simulink model "mtv1"  (R2015b)
settings: Solver=FixedStepDiscrete  SolverMode=SingleTasking  StartTime=0.0  StopTime=sim_stop_time  FixedStep=sim_time_step_size  RelTol=1e-3
PreLoadFcn:
  | nimbus_bus_all;
  | mtv_bus_all;
undefined symbols (not defined in the file or in its folder): csc_sim_mtv_simulation, csc_sim_mtv_simulation_lib, csci_gsse_mtv, csci_gsse_mtv_lib, csu_tfm_tether_mtv, ini_epoch_seconds, sim_time_step_size, swm_num_switches, tfm_attachment_location_body, tfm_cg_enable, tfm_forces_enable, tfm_hanging_location_topo, tfm_horseshoe_bolt_mass, tfm_moments_enable, tfm_sleeve_mass, tfm_tether_mass_per_length, tfm_tether_spring_constant, tfm_tether_unstretched_length
libraries: util_common_lib x8, util_info_lib x2, simulink x2, util_quat_lib x2, csci_fsw_mtv_lib x1, csc_gnd_sta_lib x1, telem_conversion_lib x1, csc_egt_egc_thruster_lib x1, csc_enf_environmental_forces_mtv_lib x1, csc_prs_pressure_system_sim_lib x1, csc_pwr_power_system_sim_lib x1, csc_rigid_body_dynamics_lib x1
settings Model: ExtModeTrigDuration=100  Creator=ianmga  LastModifiedBy=jimkaidy
settings DataIOCC: LimitDataPoints=off  SaveFormat=Array  SaveOutput=off  SaveTime=off  StateSaveName=tmp_raccel_xout  SignalLoggingName=raw_event_logs
settings OptimizationCC: ExpressionDepthLimit=2147483647  InitFltsAndDblsToZero=on  OptimizeModelRefInitCode=on
settings DebuggingCC: CheckSSInitialOutputMsg=off  UnderspecifiedInitializationDetection=Classic  MergeDetectMultiDrivingBlocksExec=none  SolverPrmCheckMsg=warning  UnderSpecifiedDataTypeMsg=warning  FcnCallInpInsideContextMsg=UseLocalSettings  BusObjectLabelMismatch=error  StateNameClashWarn=warning  StrictBusMsg=WarnOnBusTreatedAsVector
settings HardwareCC: ProdBitPerPointer=32  ProdLargestAtomicFloat=None  ProdIntDivRoundTo=Undefined  ProdEndianess=Unspecified  ProdWordSize=32  ProdHWDeviceType=32-bit Generic  TargetHWDeviceType=32-bit Generic
settings SFSimCC: SimParseCustomCode=off
settings SFSimCC: SimUserIncludeDirs=|
  | ../sim/fhw/sensors/cameras/kir
  | ../fsw/est/kcv
  | ../fsw/est/kfd
  | ../externals/minopencv/include
settings RTWCC: SystemTargetFile=ert.tlc  GenCodeOnly=on  TemplateMakefile=ert_default_tmf  Description=Embedded Coder  RetainRTWFile=on  RTWUseSimCustomCode=on
settings RTWCC: CustomInclude=|
  | ../sim/fhw/sensors/cameras/kir
  | ../fsw/est/kcv
  | ../fsw/est/kfd
  | ../externals/minopencv/include
settings CodeAppCC: ForceParamTrailComments=on  IgnoreCustomStorageClasses=off  MaxIdLength=128  SimulinkDataObjDesc=on  SFDataObjDesc=on  MangleLength=10  CustomSymbolStrType=$N$R$M  InsertBlockDesc=on  InternalIdentifier=Classic  ReqsInCode=on
settings ERTTargetCC: GenerateSampleERTMain=on  MultiInstanceERTCode=on  CodeInterfacePackaging=Reusable function  RootIOFormat=Structure reference  ERTCustomFileTemplate=csl_interface.tlc
settings ConfigComp: CovModelRefEnable=Off  CovSFcnEnable=off

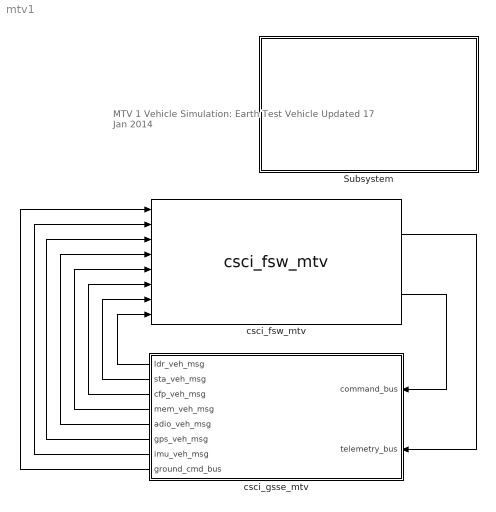
== system mtv1 ==
  note: MTV 1 Vehicle Simulation: Earth Test Vehicle
      |
      | Updated 17 Jan 2014
  Subsystem : Subsystem
      mask Display: image('nimbus2.png')
  csci_fsw_mtv : csci_fsw_mtv_lib/csci_fsw_mtv
  csci_gsse_mtv : Subsystem  AncestorBlock=csci_gsse_mtv_lib/csci_gsse_mtv
  wires:
  csci_fsw_mtv/1 -> csci_gsse_mtv/2(telemetry_bus)
  csci_gsse_mtv/2(sta_veh_msg) -> csci_fsw_mtv/7
  csci_fsw_mtv/2 -> csci_gsse_mtv/1(command_bus)
  csci_gsse_mtv/1(ldr_veh_msg) -> csci_fsw_mtv/8
  csci_gsse_mtv/3(cfp_veh_msg) -> csci_fsw_mtv/6
  csci_gsse_mtv/4(mem_veh_msg) -> csci_fsw_mtv/5
  csci_gsse_mtv/5(adio_veh_msg) -> csci_fsw_mtv/4
  csci_gsse_mtv/6(gps_veh_msg) -> csci_fsw_mtv/3
  csci_gsse_mtv/8(ground_cmd_bus) -> csci_fsw_mtv/1
  csci_gsse_mtv/7(imu_veh_msg) -> csci_fsw_mtv/2

== system mtv1/Subsystem ==

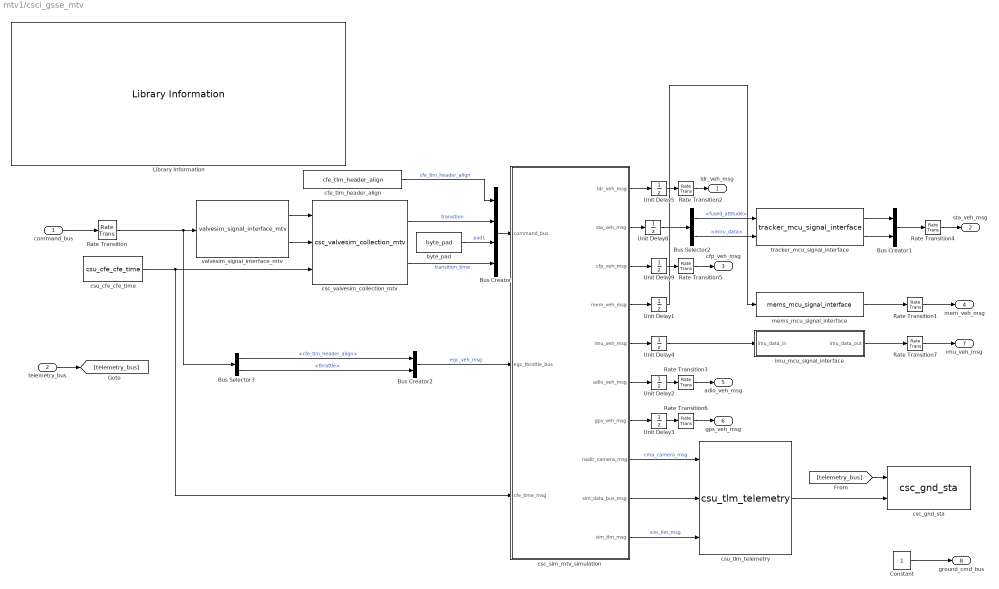
== system mtv1/csci_gsse_mtv ==
  command_bus : Inport
  telemetry_bus : Inport  Port=2
  Bus Creator : BusCreator  Inputs=4  OutDataTypeStr=Bus: thr_sim_msg  NonVirtualBus=on
  Bus Creator2 : BusCreator  Inputs=2  OutDataTypeStr=Bus: egc_veh_msg  NonVirtualBus=on
  Bus Selector2 : BusSelector  OutputSignals=fused_attitude,miru_data
  Bus Selector3 : BusSelector  OutputSignals=egc_bus_msg.cfe_tlm_header_align,egc_bus_msg.throttle
  Bus Creator1 : BusCreator  Inputs=2
  Constant : Constant
  Library Information : util_info_lib/Library Information  owner='NONE'
  Rate Transition{,1..7} (8 alike) : RateTransition  Integrity=off
  Unit Delay{1..5,8..9} (7 alike) : UnitDelay  SampleTime=-1
  byte_pad : util_common_lib/byte_pad  n_bytes=6
  cfe_tlm_header_align : util_common_lib/cfe_tlm_header_align
  csc_gnd_sta : csc_gnd_sta_lib/csc_gnd_sta  dir_name=scenario_data_dir
  csc_sim_mtv_simulation : Subsystem  Tag=GSSE; MDL_TICK=THR_SIM_MSG  AncestorBlock=csc_sim_mtv_simulation_lib/csc_sim_mtv_simulation  TreatAsAtomicUnit=on  SystemSampleTime=sim_time_step_size
  csc_valvesim_collection_mtv : csc_valvesim_collection_mtv_lib/csc_valvesim_collection_mtv  SystemSampleTime=-1
  csu_cfe_cfe_time : csu_cfe_cfe_time_lib/csu_cfe_cfe_time  sch_dt=sim_time_step_size
  csu_tlm_telemetry : csu_tlm_telemetry_lib/csu_tlm_telemetry  num_inputs=3  output_bus_name=sim_telemetry_bus_msg
  imu_mcu_signal_interface : Subsystem
  mems_mcu_signal_interface : csu_mems_mcu_signal_interface_lib/mems_mcu_signal_interface
  tracker_mcu_signal_interface : csu_tracker_mcu_signal_interface_lib/tracker_mcu_signal_interface
  valvesim_signal_interface_mtv : csu_valvesim_signal_interface_mtv_lib/valvesim_signal_interface_mtv
  ldr_veh_msg : Outport
  sta_veh_msg : Outport  Port=2
  cfp_veh_msg : Outport  Port=3
  mem_veh_msg : Outport  Port=4
  adio_veh_msg : Outport  Port=5
  gps_veh_msg : Outport  Port=6
  imu_veh_msg : Outport  Port=7
  ground_cmd_bus : Outport  Port=8
  wires:
  telemetry_bus/1 -> [telemetry_bus]
  csc_sim_mtv_simulation/9(sim_data_bus_msg) -> csu_tlm_telemetry/2
  Unit Delay9/1 -> Rate Transition5/1
  Unit Delay5/1 -> Rate Transition2/1
  csc_sim_mtv_simulation/1(ldr_veh_msg) -> Unit Delay5/1
  csc_sim_mtv_simulation/3(cfp_veh_msg) -> Unit Delay9/1
  Constant/1 -> ground_cmd_bus/1
  command_bus/1 -> Rate Transition/1
  Rate Transition2/1 -> ldr_veh_msg/1
  Rate Transition4/1 -> sta_veh_msg/1
  Rate Transition5/1 -> cfp_veh_msg/1
  csc_sim_mtv_simulation/2(sta_veh_msg) -> Unit Delay8/1
  csc_sim_mtv_simulation/8(nadir_camera_msg) -> csu_tlm_telemetry/1  "cma_camera_msg"
  csc_sim_mtv_simulation/10(sim_tlm_msg) -> csu_tlm_telemetry/3  "sim_tlm_msg"
  csu_tlm_telemetry/1 -> csc_gnd_sta/2
  [telemetry_bus] -> csc_gnd_sta/1
  valvesim_signal_interface_mtv/1 -> csc_valvesim_collection_mtv/1
  csc_valvesim_collection_mtv/1 -> Bus Creator/2  "transition"
  csc_valvesim_collection_mtv/2 -> Bus Creator/4  "transition_time"
  Bus Creator/1 -> csc_sim_mtv_simulation/1(command_bus)
  csu_cfe_cfe_time/1 -> csc_sim_mtv_simulation/3(cfe_time_msg), csc_valvesim_collection_mtv/3
  byte_pad/1 -> Bus Creator/3  "pad1"
  Rate Transition/1 -> Bus Selector3/1, valvesim_signal_interface_mtv/1
  Bus Creator2/1 -> csc_sim_mtv_simulation/2(egc_throttle_bus)  "egc_veh_msg"
  cfe_tlm_header_align/1 -> Bus Creator/1  "cfe_tlm_header_align"
  valvesim_signal_interface_mtv/2 -> csc_valvesim_collection_mtv/2
  Bus Creator1/1 -> Rate Transition4/1
  tracker_mcu_signal_interface/2 -> Bus Creator1/2
  tracker_mcu_signal_interface/1 -> Bus Creator1/1
  Bus Selector2/2 -> tracker_mcu_signal_interface/2  "<miru_data>"
  Bus Selector2/1 -> tracker_mcu_signal_interface/1  "<fused_attitude>"
  Unit Delay8/1 -> Bus Selector2/1
  csc_sim_mtv_simulation/4(mem_veh_msg) -> Unit Delay1/1
  Unit Delay1/1 -> mems_mcu_signal_interface/1
  Rate Transition1/1 -> mem_veh_msg/1
  mems_mcu_signal_interface/1 -> Rate Transition1/1
  Bus Selector3/1 -> Bus Creator2/1  "<cfe_tlm_header_align>"
  Bus Selector3/2 -> Bus Creator2/2  "<throttle>"
  Unit Delay2/1 -> Rate Transition3/1
  csc_sim_mtv_simulation/6(adio_veh_msg) -> Unit Delay2/1
  Rate Transition3/1 -> adio_veh_msg/1
  Unit Delay3/1 -> Rate Transition6/1
  Rate Transition6/1 -> gps_veh_msg/1
  csc_sim_mtv_simulation/7(gps_veh_msg) -> Unit Delay3/1
  csc_sim_mtv_simulation/5(imu_veh_msg) -> Unit Delay4/1
  Unit Delay4/1 -> imu_mcu_signal_interface/1(imu_data_in)
  Rate Transition7/1 -> imu_veh_msg/1
  imu_mcu_signal_interface/1(imu_data_out) -> Rate Transition7/1

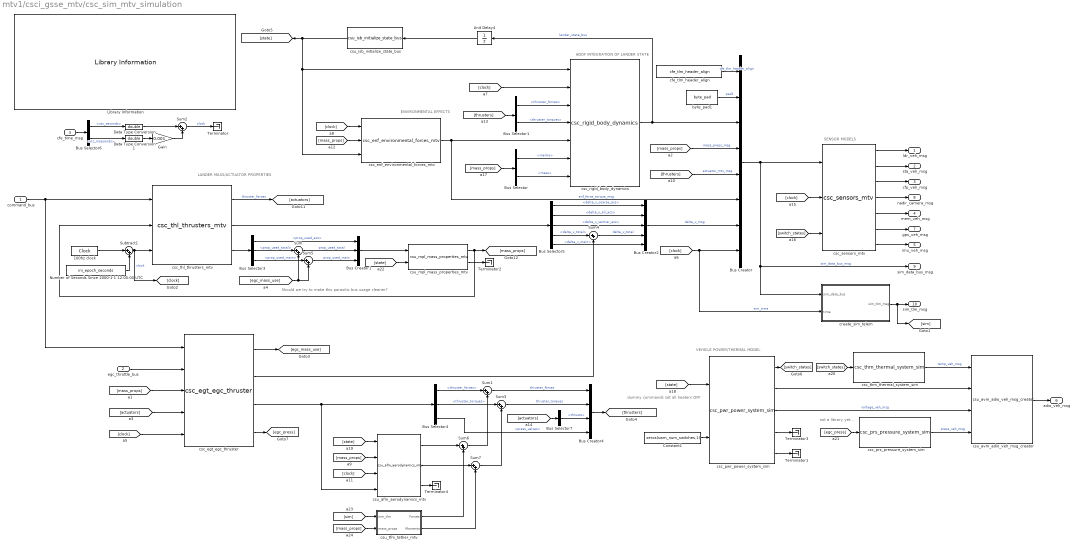
== system mtv1/csci_gsse_mtv/csc_sim_mtv_simulation ==
  note: not a library yet....
  note: VEHICLE POWER/THERMAL MODEL
  note: dummy commands set all heaters OFF
  note: LANDER MASS/ACTUATOR PROPERTIES
  note: 6DOF INTEGRATION OF LANDER STATE
  note: ENVIRONMENTAL EFFECTS
  note: SENSOR MODELS
  note: Should we try to make this parasitic bus usage cleaner?
  command_bus : Inport
  egc_throttle_bus : Inport  Port=2
  cfe_time_msg : Inport  Port=3  OutDataTypeStr=Bus: cfe_time_msg
  100hz clock : DigitalClock  SampleTime=sim_time_step_size
  Bus Creator : BusCreator  Inputs=8  OutDataTypeStr=Bus: sim_data_mtv_msg  NonVirtualBus=on
  Bus Creator1 : BusCreator  Inputs=3
  Bus Creator2 : BusCreator  Inputs=5
  Bus Creator4 : BusCreator  Inputs=4  OutDataTypeStr=Bus: actuator_mtv_msg_t
  Bus Selector : BusSelector  OutputSignals=inertia,mass
  Bus Selector1 : BusSelector  OutputSignals=thruster_forces,thruster_torques
  Bus Selector3 : BusSelector  OutputSignals=prop_used_acs,prop_used_total,prop_used_main
  Bus Selector4 : BusSelector  OutputSignals=thruster_forces,thruster_torques,press_valves
  Bus Selector5 : BusSelector  OutputSignals=delta_v_coarse_acs,delta_v_all_acs,delta_v_vernier_acs,delta_v_total,delta_v_main
  Bus Selector6 : BusSelector  OutputSignals=utc_seconds,utc_mseconds
  Bus Selector7 : BusSelector  OutputSignals=thrusts
  Constant1 : Constant  Value=zeros(swm_num_switches,1)  OutDataTypeStr=double
  Data Type Conversion : DataTypeConversion  OutDataTypeStr=double
  Data Type Conversion1 : DataTypeConversion  OutDataTypeStr=double
  Gain : Gain  Gain=0.001
  Library Information : util_info_lib/Library Information  owner='NONE'
  Number of Seconds Since 2000-1-1 12:00:00 UTC : Constant  Description=|  Value=ini_epoch_seconds
      | Number of Seconds                   
      | July 4, 2014 22:40:00 UTC           
      | Calculate on Web Site:              
      | www.mbari.org/staff/rich/utccalc.htm
  Subtract1 : Sum  Inputs=|++
  Sum{,1..7} (8 alike) : Sum  Inputs=|++
  Terminator{,1..4} (5 alike) : Terminator
  Unit Delay4 : UnitDelay  SampleTime=-1
  byte_pad1 : util_common_lib/byte_pad  n_bytes=4
  cfe_tlm_header_align : util_common_lib/cfe_tlm_header_align
  create_sim_telem : Subsystem
  csc_egt_egc_thruster : csc_egt_egc_thruster_lib/csc_egt_egc_thruster
  csc_enf_environmental_forces_mtv : csc_enf_environmental_forces_mtv_lib/csc_enf_environmental_forces_mtv
  csc_prs_pressure_system_sim : csc_prs_pressure_system_sim_lib/csc_prs_pressure_system_sim
  csc_pwr_power_system_sim : csc_pwr_power_system_sim_lib/csc_pwr_power_system_sim
  csc_rigid_body_dynamics : csc_rigid_body_dynamics_lib/csc_rigid_body_dynamics
  csc_sensors_mtv : csc_sensors_mtv_lib/csc_sensors_mtv
  csc_thl_thrusters_mtv : csc_thl_thrusters_mtv_lib/csc_thl_thrusters_mtv
  csc_thm_thermal_system_sim : csc_thm_thermal_system_sim_lib/csc_thm_thermal_system_sim
  csu_afm_aerodynamics_mtv : csu_afm_aerodynamics_lib/csu_afm_aerodynamics_mtv  SystemSampleTime=-1
  csu_avm_adio_veh_msg_creator : csu_avm_adio_veh_msg_creator_lib/csu_avm_adio_veh_msg_creator
  csu_isb_initialize_state_bus : csu_isb_initialize_state_bus_lib/csu_isb_initialize_state_bus
  csu_mpl_mass_properties_mtv : csu_mpl_mass_properties_mtv_lib/csu_mpl_mass_properties_mtv
  csu_tfm_tether_mtv : Subsystem  AncestorBlock=csu_tfm_tether_mtv/csu_tfm_tether_mtv
  ldr_veh_msg : Outport
  sta_veh_msg : Outport  Port=2
  cfp_veh_msg : Outport  Port=3
  mem_veh_msg : Outport  Port=4
  imu_veh_msg : Outport  Port=5
  adio_veh_msg : Outport  Port=6
  gps_veh_msg : Outport  Port=7
  nadir_camera_msg : Outport  Port=8
  sim_data_bus_msg : Outport  Port=9
  sim_tlm_msg : Outport  Port=10
  wires:
  csu_afm_aerodynamics_mtv/3 -> Terminator4/1
  [clock] -> csu_afm_aerodynamics_mtv/3
  Sum3/1 -> Bus Creator4/2  "thruster_torques"
  Bus Selector7/1 -> Bus Creator4/3  "<thrusts>"
  [actuators] -> Bus Selector7/1
  Bus Creator4/1 -> [thrusters]
  Sum1/1 -> Bus Creator4/1  "thruster_forces"
  csc_egt_egc_thruster/3 -> Bus Selector4/1, csu_afm_aerodynamics_mtv/4
  [switch_states] -> csc_sensors_mtv/3
  csc_pwr_power_system_sim/5 -> Terminator1/1
  csc_pwr_power_system_sim/4 -> Terminator3/1
  csc_pwr_power_system_sim/1 -> [switch_states]
  [state] -> csc_pwr_power_system_sim/1
  Constant1/1 -> csc_pwr_power_system_sim/2
  [clock] -> csc_sensors_mtv/2
  Unit Delay4/1 -> csu_isb_initialize_state_bus/1
  csu_isb_initialize_state_bus/1 -> csc_enf_environmental_forces_mtv/3, csc_rigid_body_dynamics/1, [state]
  [clock] -> csc_rigid_body_dynamics/2
  cfe_tlm_header_align/1 -> Bus Creator/1  "cfe_tlm_header_align"
  csc_sensors_mtv/4 -> nadir_camera_msg/1
  csc_sensors_mtv/3 -> cfp_veh_msg/1
  csc_sensors_mtv/2 -> sta_veh_msg/1
  csc_sensors_mtv/1 -> ldr_veh_msg/1
  Bus Selector6/1 -> Data Type Conversion/1  "<utc_seconds>"
  Gain/1 -> Sum2/2
  Data Type Conversion1/1 -> Gain/1
  Data Type Conversion/1 -> Sum2/1
  Bus Selector6/2 -> Data Type Conversion1/1  "<utc_mseconds>"
  cfe_time_msg/1 -> Bus Selector6/1
  egc_throttle_bus/1 -> csc_egt_egc_thruster/2
  [mass_props] -> csc_egt_egc_thruster/3
  [actuators] -> csc_egt_egc_thruster/4
  Bus Selector5/1 -> Bus Creator2/1  "<delta_v_coarse_acs>"
  Bus Selector5/2 -> Bus Creator2/2  "<delta_v_all_acs>"
  Bus Selector5/3 -> Bus Creator2/3  "<delta_v_vernier_acs>"
  Bus Selector5/5 -> Bus Creator2/5  "<delta_v_main>"
  Sum4/1 -> Bus Creator2/4  "delta_v_total"
  Bus Selector5/4 -> Sum4/1  "<delta_v_total>"
  csc_thl_thrusters_mtv/2 -> Bus Selector5/1
  Bus Creator2/1 -> Bus Creator/7  "delta_v_msg"
  csc_egt_egc_thruster/2 -> Sum4/2
  Bus Creator1/1 -> csu_mpl_mass_properties_mtv/1
  Bus Selector3/3 -> Sum5/1  "<prop_used_main>"
  Bus Selector3/1 -> Bus Creator1/1  "<prop_used_acs>"
  Sum/1 -> Bus Creator1/2  "prop_used_total"
  [egc_mass_use] -> Sum5/2, Sum/2
  Bus Selector3/2 -> Sum/1  "<prop_used_total>"
  csc_egt_egc_thruster/1 -> [egc_mass_use]
  csc_thl_thrusters_mtv/3 -> Bus Selector3/1
  byte_pad1/1 -> Bus Creator/2  "pad1"
  Subtract1/1 -> [clock], csc_thl_thrusters_mtv/3  "clock"
  [clock] -> Bus Creator/8, create_sim_telem/2(time)  "sim_time"
  create_sim_telem/1(sim_tlm_msg) -> [sim], sim_tlm_msg/1
  Bus Creator/1 -> create_sim_telem/1(sim_data_bus), sim_data_bus_msg/1, csc_sensors_mtv/1  "sim_data_bus_msg"
  csc_rigid_body_dynamics/1 -> Unit Delay4/1, Bus Creator/3  "lander_state_bus"
  [mass_props] -> Bus Selector/1
  [thrusters] -> Bus Selector1/1
  [thrusters] -> Bus Creator/5  "actuator_mtv_msg"
  [mass_props] -> Bus Creator/4  "mass_props_msg"
  Bus Selector/2 -> csc_rigid_body_dynamics/7  "<mass>"
  Bus Selector/1 -> csc_rigid_body_dynamics/6  "<inertia>"
  csu_mpl_mass_properties_mtv/1 -> csc_thl_thrusters_mtv/2, [mass_props]
  Bus Selector1/1 -> csc_rigid_body_dynamics/3  "<thruster_forces>"
  Bus Selector1/2 -> csc_rigid_body_dynamics/4  "<thruster_torques>"
  csc_enf_environmental_forces_mtv/1 -> csc_rigid_body_dynamics/5, Bus Creator/6  "enf_force_torque_msg"
  csc_thl_thrusters_mtv/1 -> [actuators]  "thruster_forces"
  [clock] -> csc_enf_environmental_forces_mtv/1
  [mass_props] -> csc_enf_environmental_forces_mtv/2
  csc_sensors_mtv/5 -> mem_veh_msg/1
  Number of Seconds Since 2000-1-1 12:00:00 UTC/1 -> Subtract1/2
  100hz clock/1 -> Subtract1/1
  Sum2/1 -> Terminator/1  "clock"
  [switch_states] -> csc_thm_thermal_system_sim/1
  csu_avm_adio_veh_msg_creator/1 -> adio_veh_msg/1
  csc_thm_thermal_system_sim/1 -> csu_avm_adio_veh_msg_creator/1  "temp_veh_msg"
  csc_pwr_power_system_sim/2 -> csu_avm_adio_veh_msg_creator/2
  csc_pwr_power_system_sim/3 -> csu_avm_adio_veh_msg_creator/3  "voltage_veh_msg"
  [egc_press] -> csc_prs_pressure_system_sim/1
  csc_prs_pressure_system_sim/1 -> csu_avm_adio_veh_msg_creator/4  "press_veh_msg"
  csc_egt_egc_thruster/4 -> [egc_press]
  command_bus/1 -> csc_egt_egc_thruster/1, csc_thl_thrusters_mtv/1
  [clock] -> csc_egt_egc_thruster/5
  Sum5/1 -> Bus Creator1/3  "prop_used_main"
  Bus Selector4/3 -> Bus Creator4/4  "<press_valves>"
  csu_mpl_mass_properties_mtv/2 -> Terminator2/1
  csc_sensors_mtv/6 -> gps_veh_msg/1
  [state] -> csu_mpl_mass_properties_mtv/2
  csc_sensors_mtv/7 -> imu_veh_msg/1
  [mass_props] -> csu_afm_aerodynamics_mtv/2
  [state] -> csu_afm_aerodynamics_mtv/1
  Bus Selector4/1 -> Sum1/1  "<thruster_forces>"
  Bus Selector4/2 -> Sum3/1  "<thruster_torques>"
  [mass_props] -> csu_tfm_tether_mtv/2(mass_props)
  [sim] -> csu_tfm_tether_mtv/1(sim_tlm)
  csu_afm_aerodynamics_mtv/1 -> Sum6/1
  csu_tfm_tether_mtv/1(Forces) -> Sum6/2
  csu_afm_aerodynamics_mtv/2 -> Sum7/1
  csu_tfm_tether_mtv/2(Moments) -> Sum7/2
  Sum6/1 -> Sum1/2
  Sum7/1 -> Sum3/2

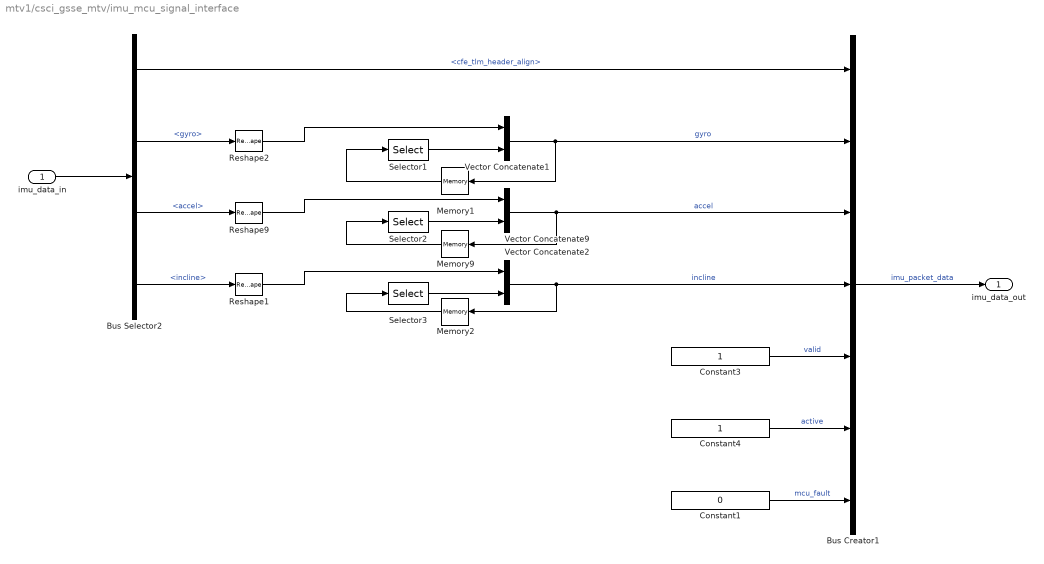
== system mtv1/csci_gsse_mtv/imu_mcu_signal_interface ==
  imu_data_in : Inport
  Bus Selector2 : BusSelector  OutputSignals=cfe_tlm_header_align,gyro,accel,incline
  Bus Creator1 : BusCreator  Inputs=7
  Constant1 : Constant  Value=0  OutDataTypeStr=uint8
  Constant3 : Constant  OutDataTypeStr=uint16
  Constant4 : Constant  OutDataTypeStr=uint8
  Memory1 : Memory  X0=zeros(10,3)  InheritSampleTime=on
  Memory2 : Memory  X0=zeros(10,3)  InheritSampleTime=on
  Memory9 : Memory  X0=zeros(10,3)  InheritSampleTime=on
  Reshape1 : Reshape  OutputDimensionality=Row vector (2-D)
  Reshape2 : Reshape  OutputDimensionality=Row vector (2-D)
  Reshape9 : Reshape  OutputDimensionality=Row vector (2-D)
  Selector1 : Selector  NumberOfDimensions=2  InputPortWidth=10  IndexOptions=Index vector (dialog),Select all  Indices=[1:9],1  OutputSizes=1,1
  Selector2 : Selector  NumberOfDimensions=2  InputPortWidth=10  IndexOptions=Index vector (dialog),Select all  Indices=[1:9],1  OutputSizes=1,1
  Selector3 : Selector  NumberOfDimensions=2  InputPortWidth=10  IndexOptions=Index vector (dialog),Select all  Indices=[1:9],1  OutputSizes=1,1
  Vector Concatenate1 : Concatenate  Mode=Multidimensional array
  Vector Concatenate2 : Concatenate  Mode=Multidimensional array
  Vector Concatenate9 : Concatenate  Mode=Multidimensional array
  imu_data_out : Outport
  wires:
  Bus Selector2/4 -> Reshape1/1  "<incline>"
  Memory2/1 -> Selector3/1
  Selector3/1 -> Vector Concatenate2/2
  Vector Concatenate2/1 -> Bus Creator1/4, Memory2/1  "incline"
  Reshape1/1 -> Vector Concatenate2/1
  Bus Selector2/1 -> Bus Creator1/1  "<cfe_tlm_header_align>"
  Bus Creator1/1 -> imu_data_out/1  "imu_packet_data"
  imu_data_in/1 -> Bus Selector2/1
  Memory1/1 -> Selector1/1
  Selector1/1 -> Vector Concatenate1/2
  Vector Concatenate1/1 -> Memory1/1, Bus Creator1/2  "gyro"
  Reshape2/1 -> Vector Concatenate1/1
  Memory9/1 -> Selector2/1
  Selector2/1 -> Vector Concatenate9/2
  Vector Concatenate9/1 -> Bus Creator1/3, Memory9/1  "accel"
  Reshape9/1 -> Vector Concatenate9/1
  Constant3/1 -> Bus Creator1/5  "valid"
  Constant4/1 -> Bus Creator1/6  "active"
  Constant1/1 -> Bus Creator1/7  "mcu_fault"
  Bus Selector2/2 -> Reshape2/1  "<gyro>"
  Bus Selector2/3 -> Reshape9/1  "<accel>"

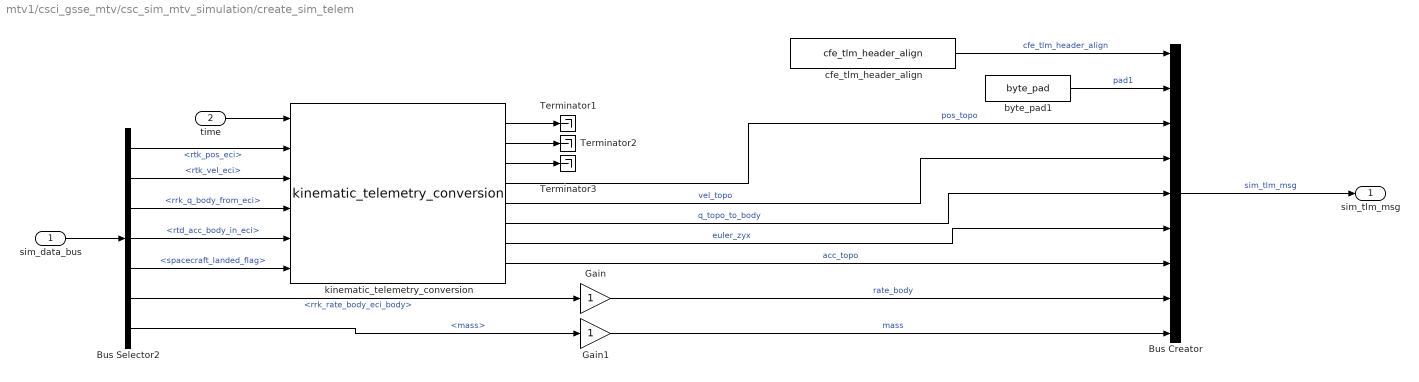
== system mtv1/csci_gsse_mtv/csc_sim_mtv_simulation/create_sim_telem ==
  sim_data_bus : Inport
  time : Inport  Port=2
  Bus Creator : BusCreator  Inputs=9  OutDataTypeStr=Bus: sim_tlm_msg  NonVirtualBus=on
  Bus Selector2 : BusSelector  OutputSignals=lander_state_bus.rtk_pos_eci,lander_state_bus.rtk_vel_eci,lander_state_bus.rrk_q_body_from_eci,lander_state_bus.rtd_acc_body_in_eci,lander_state_bus.spacecraft_landed_flag,lander_state_bus.rrk_rate_body_eci_body,mass_props_msg.mass
  Gain : Gain
  Gain1 : Gain
  Terminator1 : Terminator
  Terminator2 : Terminator
  Terminator3 : Terminator
  byte_pad1 : util_common_lib/byte_pad  n_bytes=4
  cfe_tlm_header_align : util_common_lib/cfe_tlm_header_align
  kinematic_telemetry_conversion : telem_conversion_lib/kinematic_telemetry_conversion
  sim_tlm_msg : Outport
  wires:
  cfe_tlm_header_align/1 -> Bus Creator/1  "cfe_tlm_header_align"
  byte_pad1/1 -> Bus Creator/2  "pad1"
  kinematic_telemetry_conversion/3 -> Terminator3/1
  kinematic_telemetry_conversion/2 -> Terminator2/1
  kinematic_telemetry_conversion/1 -> Terminator1/1
  Bus Creator/1 -> sim_tlm_msg/1  "sim_tlm_msg"
  kinematic_telemetry_conversion/8 -> Bus Creator/7  "acc_topo"
  kinematic_telemetry_conversion/7 -> Bus Creator/6  "euler_zyx"
  kinematic_telemetry_conversion/6 -> Bus Creator/5  "q_topo_to_body"
  kinematic_telemetry_conversion/5 -> Bus Creator/4  "vel_topo"
  sim_data_bus/1 -> Bus Selector2/1
  time/1 -> kinematic_telemetry_conversion/1
  Bus Selector2/1 -> kinematic_telemetry_conversion/2  "<rtk_pos_eci>"
  Bus Selector2/2 -> kinematic_telemetry_conversion/3  "<rtk_vel_eci>"
  Bus Selector2/3 -> kinematic_telemetry_conversion/4  "<rrk_q_body_from_eci>"
  Bus Selector2/4 -> kinematic_telemetry_conversion/5  "<rtd_acc_body_in_eci>"
  Bus Selector2/6 -> Gain/1  "<rrk_rate_body_eci_body>"
  Gain/1 -> Bus Creator/8  "rate_body"
  Bus Selector2/7 -> Gain1/1  "<mass>"
  Gain1/1 -> Bus Creator/9  "mass"
  kinematic_telemetry_conversion/4 -> Bus Creator/3  "pos_topo"
  Bus Selector2/5 -> kinematic_telemetry_conversion/6  "<spacecraft_landed_flag>"

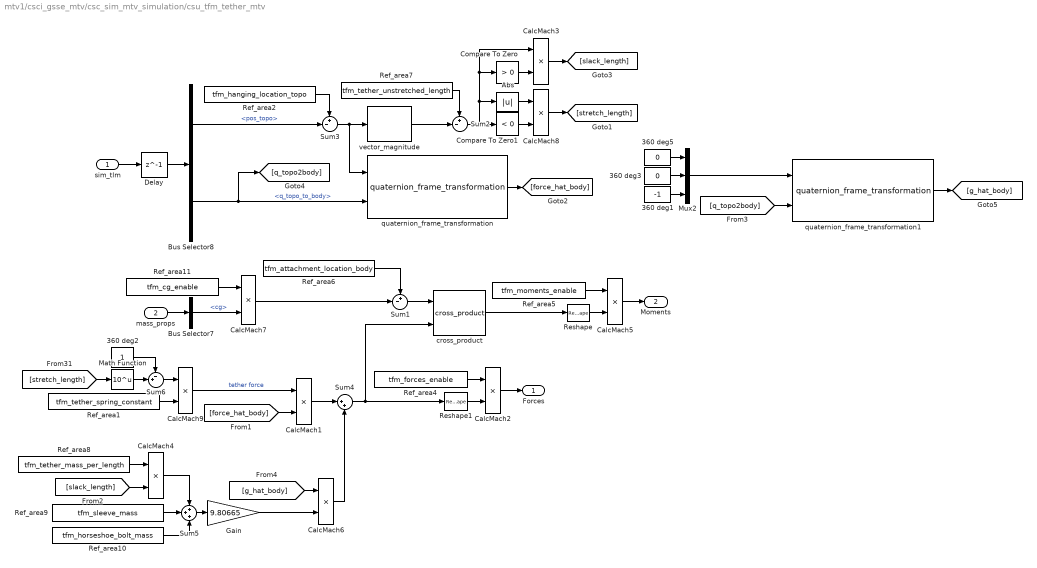
== system mtv1/csci_gsse_mtv/csc_sim_mtv_simulation/csu_tfm_tether_mtv ==
  sim_tlm : Inport
  mass_props : Inport  Port=2
  360 deg1 : Constant  Value=-1
  360 deg2 : Constant
  360 deg3 : Constant  Value=0
  360 deg5 : Constant  Value=0
  Abs : Abs
  Bus Selector7 : BusSelector  OutputSignals=cg
  Bus Selector8 : BusSelector  OutputSignals=pos_topo,q_topo_to_body
  CalcMach{1..9} (9 alike) : Product  SaturateOnIntegerOverflow=on  OutDataTypeStr=Inherit: Same as first input
  Compare To Zero : simulink/Logic and Bit Operations/Compare To Zero  relop=>  OutDataTypeStr=uint8
  Compare To Zero1 : simulink/Logic and Bit Operations/Compare To Zero  relop=<  OutDataTypeStr=uint8
  Delay : Delay  DelayLength=1
  Gain : Gain  Gain=9.80665
  Math Function : Math  Operator=10^u  SaturateOnIntegerOverflow=on
  Mux2 : Mux  Inputs=3
  Ref_area1 : Constant  Value=tfm_tether_spring_constant
  Ref_area10 : Constant  Value=tfm_horseshoe_bolt_mass
  Ref_area11 : Constant  Value=tfm_cg_enable
  Ref_area2 : Constant  Value=tfm_hanging_location_topo
  Ref_area4 : Constant  Value=tfm_forces_enable
  Ref_area5 : Constant  Value=tfm_moments_enable
  Ref_area6 : Constant  Value=tfm_attachment_location_body
  Ref_area7 : Constant  Value=tfm_tether_unstretched_length
  Ref_area8 : Constant  Value=tfm_tether_mass_per_length
  Ref_area9 : Constant  Value=tfm_sleeve_mass
  Reshape : Reshape
  Reshape1 : Reshape
  Sum1 : Sum  Inputs=+-|
  Sum2 : Sum  Inputs=+-|
  Sum3 : Sum  Inputs=+-|
  Sum4 : Sum  Inputs=|++
  Sum5 : Sum  Inputs=+++
  Sum6 : Sum  Inputs=-+|
  cross_product : util_common_lib/cross_product  SystemSampleTime=-1
  quaternion_frame_transformation : util_quat_lib/quaternion_frame_transformation  SystemSampleTime=-1
  quaternion_frame_transformation1 : util_quat_lib/quaternion_frame_transformation  SystemSampleTime=-1
  vector_magnitude : util_common_lib/vector_magnitude  SystemSampleTime=-1
  Forces : Outport
  Moments : Outport  Port=2
  wires:
  Gain/1 -> CalcMach6/2
  Sum3/1 -> vector_magnitude/1, quaternion_frame_transformation/1
  CalcMach3/1 -> [slack_length]
  Sum2/1 -> CalcMach3/1, Compare To Zero/1, Abs/1, Compare To Zero1/1
  Ref_area7/1 -> Sum2/1
  cross_product/1 -> Reshape/1
  Ref_area5/1 -> CalcMach5/1
  Sum1/1 -> cross_product/1
  Ref_area6/1 -> Sum1/1
  CalcMach5/1 -> Moments/1
  CalcMach9/1 -> CalcMach1/1  "tether force"
  [force_hat_body] -> CalcMach1/2
  CalcMach2/1 -> Forces/1
  Ref_area4/1 -> CalcMach2/1
  quaternion_frame_transformation/1 -> [force_hat_body]
  Bus Selector8/2 -> quaternion_frame_transformation/2, [q_topo2body]  "<q_topo_to_body>"
  Ref_area1/1 -> CalcMach9/2
  [stretch_length] -> Math Function/1
  Ref_area2/1 -> Sum3/1
  vector_magnitude/1 -> Sum2/2
  Bus Selector8/1 -> Sum3/2  "<pos_topo>"
  mass_props/1 -> Bus Selector7/1
  Mux2/1 -> quaternion_frame_transformation1/1
  360 deg3/1 -> Mux2/2
  360 deg5/1 -> Mux2/1
  [q_topo2body] -> quaternion_frame_transformation1/2
  Ref_area8/1 -> CalcMach4/1
  360 deg1/1 -> Mux2/3
  quaternion_frame_transformation1/1 -> [g_hat_body]
  [g_hat_body] -> CalcMach6/1
  [slack_length] -> CalcMach4/2
  Sum4/1 -> Reshape1/1, cross_product/2
  Ref_area9/1 -> Sum5/2
  CalcMach4/1 -> Sum5/1
  Ref_area10/1 -> Sum5/3
  Sum5/1 -> Gain/1
  Reshape/1 -> CalcMach5/2
  Reshape1/1 -> CalcMach2/2
  sim_tlm/1 -> Delay/1
  Delay/1 -> Bus Selector8/1
  Ref_area11/1 -> CalcMach7/1
  Bus Selector7/1 -> CalcMach7/2  "<cg>"
  CalcMach7/1 -> Sum1/2
  Math Function/1 -> Sum6/2
  CalcMach8/1 -> [stretch_length]
  Compare To Zero/1 -> CalcMach3/2
  Compare To Zero1/1 -> CalcMach8/2
  Abs/1 -> CalcMach8/1
  CalcMach1/1 -> Sum4/1
  CalcMach6/1 -> Sum4/2
  Sum6/1 -> CalcMach9/1
  360 deg2/1 -> Sum6/1
